simulink model "sigma_delta_2nd_ordre_z"  (Simulink 6.2)
settings: Solver=ode3  StartTime=0.0  StopTime=1-1/fck  FixedStep=1/fck  RelTol=1e-3
values from neighbouring files (symbols this model uses):
  B = 3    [main_sigma_delta.m]
  fck = 1000000    [main_sigma_delta.m]
  noise_2 = 0    [main_sigma_delta.m]
  tau = 1/(2*pi*fc)    (= 0.0159154943092)    [main_sigma_delta.m]
libraries: simulink x1
settings Model: LastModifiedBy=Mailly
settings DebuggingCC: SolverPrmCheckMsg=warning

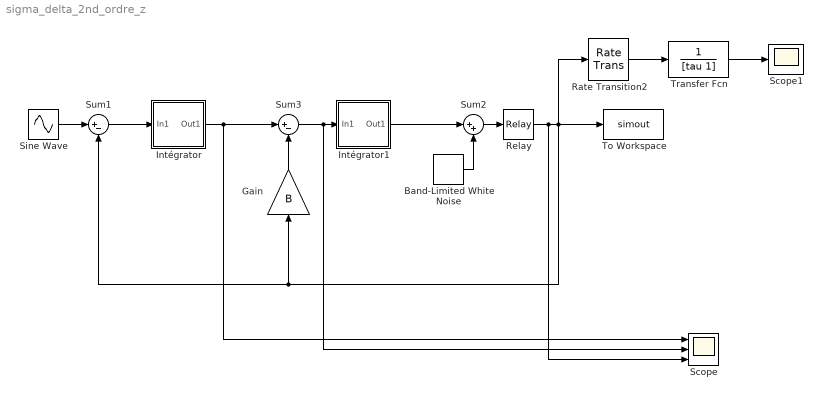
== system sigma_delta_2nd_ordre_z ==
  Band-Limited White Noise : simulink/Sources/Band-Limited White Noise  Cov=[noise_2]  Ts=1/fck  seed=[23341]
  Gain : Gain  Orientation=up  Gain=B
  Intégrator : Subsystem
  Intégrator1 : Subsystem
  Rate Transition2 : RateTransition
  Relay : Relay  OnSwitchValue=0  OffSwitchValue=0  OffOutputValue=-1  SampleTime=1/fck
  Scope : Scope  NumInputPorts=3
      settings: YMin=-0.0025~-2~-1750  YMax=0.03~2~1500
  Scope1 : Scope
      settings: YMin=-1  YMax=1
  Sine Wave : Sin  Amplitude=0.5  Frequency=2*pi*10  SampleTime=1/fck
  Sum1 : Sum  Inputs=|+-
  Sum2 : Sum  Inputs=|++
  Sum3 : Sum  Inputs=|+-
  To Workspace : ToWorkspace  VariableName=simout  SampleTime=1/fck  SaveFormat=Array
      settings: MaxDataPoints=fck
  Transfer Fcn : TransferFcn  Denominator=[tau 1]
  wires:
  Sine Wave/1 -> Sum1/1
  Sum1/1 -> Intégrator/1(In1)
  Relay/1 -> To Workspace/1, Rate Transition2/1, Sum1/2, Gain/1, Scope/3
  Band-Limited White Noise/1 -> Sum2/2
  Transfer Fcn/1 -> Scope1/1
  Rate Transition2/1 -> Transfer Fcn/1
  Intégrator/1(Out1) -> Scope/1, Sum3/1
  Sum2/1 -> Relay/1
  Sum3/1 -> Intégrator1/1(In1), Scope/2
  Intégrator1/1(Out1) -> Sum2/1
  Gain/1 -> Sum3/2

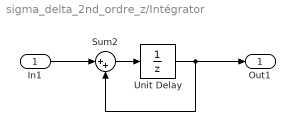
== system sigma_delta_2nd_ordre_z/Intégrator ==
  In1 : Inport  Port=1  LatchInput=off
  Sum2 : Sum  Inputs=|++
  Unit Delay : UnitDelay  SampleTime=1/fck
  Out1 : Outport
  wires:
  In1/1 -> Sum2/1
  Sum2/1 -> Unit Delay/1
  Unit Delay/1 -> Out1/1, Sum2/2

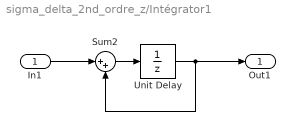
== system sigma_delta_2nd_ordre_z/Intégrator1 ==
  In1 : Inport  Port=1  LatchInput=off
  Sum2 : Sum  Inputs=|++
  Unit Delay : UnitDelay  SampleTime=1/fck
  Out1 : Outport
  wires:
  In1/1 -> Sum2/1
  Sum2/1 -> Unit Delay/1
  Unit Delay/1 -> Out1/1, Sum2/2
